simulink model "Subsystem10"  (R2020b)
settings: Solver=FixedStepAuto  StartTime=0.0  StopTime=10.0  FixedStep=0.001  RelTol=1e-3
values from neighbouring files (symbols this model uses):
  b0 = 1    [Initialization.m]
  b1 = 2    [Initialization.m]
  b2 = -3    [Initialization.m]
  b3 = -4    [Initialization.m]
  b4 = 5    [Initialization.m]
settings Model: Creator=Lakshmi  LastModifiedBy=Lakshmi
settings DataIOCC: SaveOutput=off  SaveTime=off

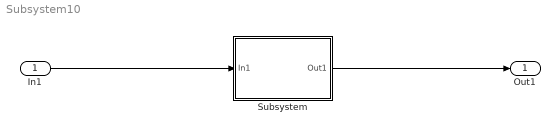
== system Subsystem10 ==
  In1 : Inport  OutDataTypeStr=double  PortDimensions=1  SampleTime=0
  Subsystem : Subsystem
  Out1 : Outport  OutDataTypeStr=double  PortDimensions=1  SampleTime=0
  wires:
  In1/1 -> Subsystem/1(In1)
  Subsystem/1(Out1) -> Out1/1

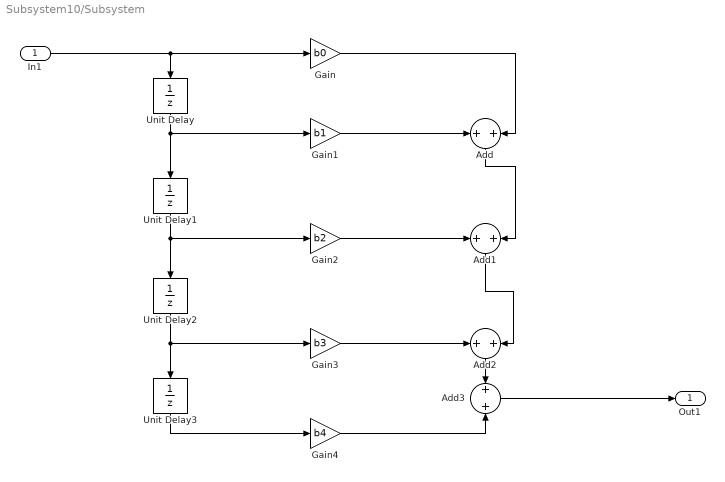
== system Subsystem10/Subsystem ==
  In1 : Inport
  Add{,1..3} (4 alike) : Sum
  Gain : Gain  Gain=b0
  Gain1 : Gain  Gain=b1
  Gain2 : Gain  Gain=b2
  Gain3 : Gain  Gain=b3
  Gain4 : Gain  Gain=b4
  Unit Delay{,1..3} (4 alike) : UnitDelay  SampleTime=-1  HasFrameUpgradeWarning=on
  Out1 : Outport
  wires:
  Add3/1 -> Out1/1
  Gain1/1 -> Add/1
  Gain4/1 -> Add3/2
  Add2/1 -> Add3/1
  Add1/1 -> Add2/2
  Unit Delay1/1 -> Unit Delay2/1, Gain2/1
  Add/1 -> Add1/2
  Unit Delay3/1 -> Gain4/1
  Gain/1 -> Add/2
  In1/1 -> Unit Delay/1, Gain/1
  Gain3/1 -> Add2/1
  Gain2/1 -> Add1/1
  Unit Delay/1 -> Unit Delay1/1, Gain1/1
  Unit Delay2/1 -> Gain3/1, Unit Delay3/1
